simulink model "wariant2"  (R2016b)
settings: Solver=VariableStepAuto  StartTime=0.0  StopTime=10.0  RelTol=1e-3
settings Model: Creator=E7440  LastModifiedBy=E7440

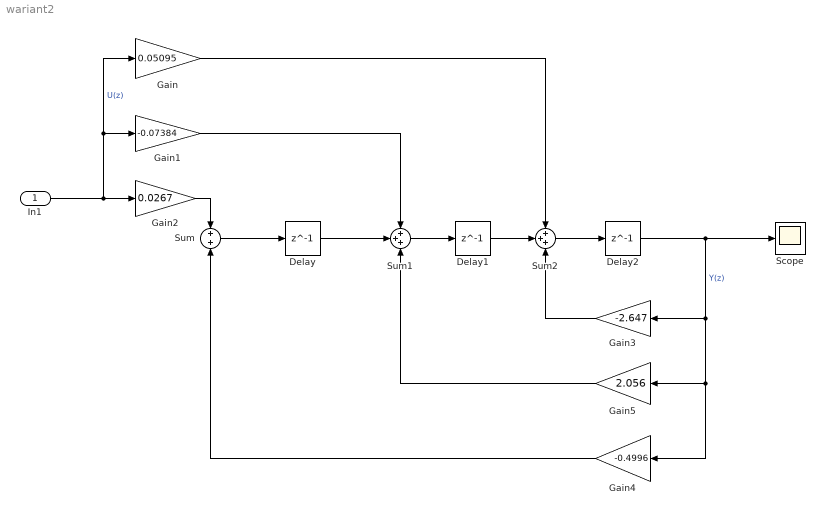
== system wariant2 ==
  In1 : Inport
  Delay : Delay  DelayLength=1  InitialCondition=3
  Delay1 : Delay  DelayLength=1  InitialCondition=-1
  Delay2 : Delay  DelayLength=1  InitialCondition=1
  Gain : Gain  Gain=0.05095
  Gain1 : Gain  Gain=-0.07384
  Gain2 : Gain  Gain=0.0267
  Gain3 : Gain  Gain=-2.647
  Gain4 : Gain  Gain=-0.4996
  Gain5 : Gain  Gain=2.056
  Scope : Scope
  Sum : Sum
  Sum1 : Sum  Inputs=+++
  Sum2 : Sum  Inputs=+++
  wires:
  In1/1 -> Gain/1, Gain1/1, Gain2/1  "U(z)"
  Sum/1 -> Delay/1
  Gain3/1 -> Sum2/3
  Delay2/1 -> Scope/1, Gain3/1, Gain5/1, Gain4/1  "Y(z)"
  Gain2/1 -> Sum/1
  Delay1/1 -> Sum2/2
  Sum2/1 -> Delay2/1
  Delay/1 -> Sum1/2
  Sum1/1 -> Delay1/1
  Gain5/1 -> Sum1/3
  Gain4/1 -> Sum/2
  Gain/1 -> Sum2/1
  Gain1/1 -> Sum1/1
